simulink model "Lab3_controller"  (R2014a)
settings: Solver=ode45  StartTime=0.0  StopTime=1  MaxStep=.001  RelTol=1e-3
values from neighbouring files (symbols this model uses):
  K = 19.4    [Lab3code.m]
  K_d = 0.0318    [Lab3code.m]
  K_r = 0    [Lab3code.m]
  T_d = 1    [Lab3code.m]
settings Model: Creator=Matthew  LastModifiedBy=mmroman2
settings DataIOCC: LimitDataPoints=off

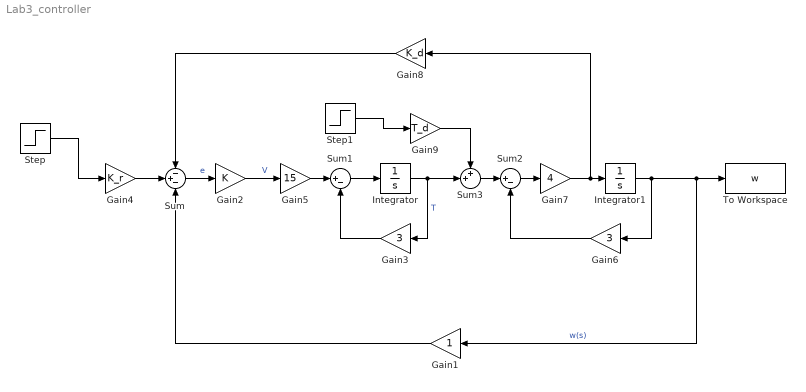
== system Lab3_controller ==
  Gain1 : Gain
  Gain2 : Gain  Gain=K
  Gain3 : Gain  Gain=3
  Gain4 : Gain  Gain=K_r
  Gain5 : Gain  Gain=15
  Gain6 : Gain  Gain=3
  Gain7 : Gain  Gain=4
  Gain8 : Gain  Gain=K_d
  Gain9 : Gain  Gain=T_d
  Integrator : Integrator
  Integrator1 : Integrator
  Step : Step  Time=0  SampleTime=0
  Step1 : Step  Time=0  SampleTime=0
  Sum : Sum  Inputs=-+-
  Sum1 : Sum  Inputs=|+-
  Sum2 : Sum  Inputs=|+-
  Sum3 : Sum  Inputs=++|
  To Workspace : ToWorkspace  VariableName=w  SampleTime=-1
  wires:
  Gain1/1 -> Sum/3
  Sum/1 -> Gain2/1  "e"
  Integrator/1 -> Gain3/1, Sum3/2  "T"
  Gain3/1 -> Sum1/2
  Gain5/1 -> Sum1/1
  Sum1/1 -> Integrator/1
  Gain2/1 -> Gain5/1  "V"
  Sum2/1 -> Gain7/1
  Gain7/1 -> Gain8/1, Integrator1/1
  Integrator1/1 -> Gain6/1, Gain1/1, To Workspace/1  "w(s)"
  Sum3/1 -> Sum2/1
  Gain6/1 -> Sum2/2
  Step/1 -> Gain4/1
  Gain8/1 -> Sum/1
  Gain4/1 -> Sum/2
  Gain9/1 -> Sum3/1
  Step1/1 -> Gain9/1
